simulink model "random_flips"  (R2021b)
settings: Solver=VariableStepAuto  StartTime=0.0  StopTime=20  RelTol=1e-3
libraries: wnnlib x3, simulink x1
settings Model: Creator=20214358  LastModifiedBy=20214358

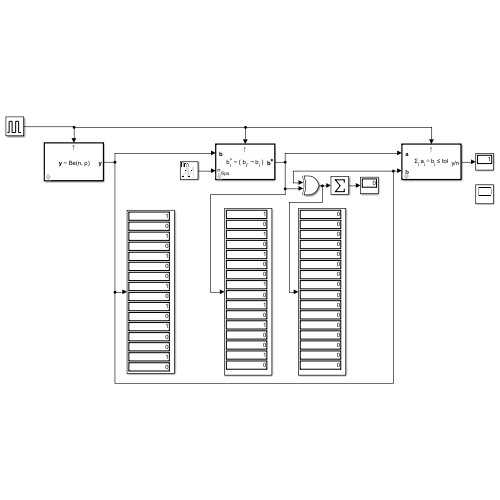
[thumbnail: Simulink's stored preview of the top-level diagram]
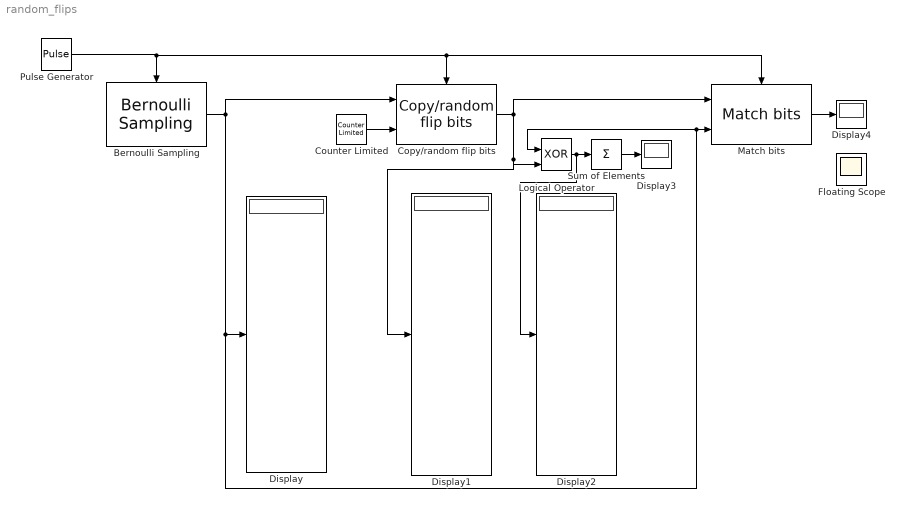
== system random_flips ==
  Bernoulli Sampling : wnnlib/Sources/Bernoulli Sampling  nSamples=16  probability=0.5  nSeed=0
      settings: SourceProductName=Weightless Neural Networks Toolbox
  Copy/random flip bits : wnnlib/Utilities/Copy//random flip bits
      settings: SourceProductName=Weightless Neural Networks Toolbox
  Counter Limited : simulink/Sources/Counter Limited  uplimit=4  tsamp=1
  Display{,1..4} (5 alike) : Display
  Floating Scope : Scope
      settings: Floating=on
  Logical Operator : Logic  Operator=XOR  IconShape=distinctive  AllPortsSameDT=off  OutDataTypeStr=boolean
  Match bits : wnnlib/Utilities/Match bits  nMatchTolerance=1
      settings: SourceProductName=Weightless Neural Networks Toolbox
  Pulse Generator : DiscretePulseGenerator  PulseType=Time based  Period=1  PulseWidth=5
  Sum of Elements : Sum  Inputs=+
  wires:
  Pulse Generator/1 -> Match bits/Trigger, Copy/random flip bits/Trigger, Bernoulli Sampling/Trigger
  Copy/random flip bits/1 -> Display1/1, Logical Operator/2, Match bits/1
  Counter Limited/1 -> Copy/random flip bits/2
  Logical Operator/1 -> Display2/1, Sum of Elements/1
  Sum of Elements/1 -> Display3/1
  Bernoulli Sampling/1 -> Match bits/2, Logical Operator/1, Display/1, Copy/random flip bits/1
  Match bits/1 -> Display4/1
